simulink model "SupervisorB1"  (R2024b)
settings: Solver=FixedStepDiscrete  StartTime=0.0  StopTime=10.0  FixedStep=0.02  RelTol=1e-3
settings Model: DataDictionary=B1Sup.sldd  PacingRate=0.100000  Creator=miche  LastModifiedBy=Sterm
settings OptimizationCC: DefaultParameterBehavior=Inlined  EnhancedBackFolding=on  PassReuseOutputArgsAs=Individual arguments  ZeroExternalMemoryAtStartup=off  ZeroInternalMemoryAtStartup=off  OptimizeBlockOrder=speed  DifferentSizesBufferReuse=on  OptimizationCustomize=off  EfficientTunableParamExpr=on
settings DebuggingCC: ParameterTunabilityLossMsg=error
settings SFSimCC: MATLABDynamicMemAlloc=off
settings SFSimCC: SimUserIncludeDirs=|
  | C:\Users\Sterm\Desktop\STM32\workspace\Codice_Rover
  | C:\Users\Sterm\Desktop\STM32\workspace\Codice_Rover\Progetto_Board1\Core\Inc
settings RTWCC: Description=Embedded Coder  SystemTargetFile=ert.tlc  GenCodeOnly=on  TemplateMakefile=ert_default_tmf
settings CodeAppCC: ForceParamTrailComments=on  IgnoreCustomStorageClasses=off  OperatorAnnotations=on  SimulinkDataObjDesc=on  SFDataObjDesc=on  InsertBlockDesc=on
settings ERTTargetCC: TargetLangStandard=C99 (ISO)  GenerateSampleERTMain=on  ERTCustomFileTemplate=example_file_process.tlc

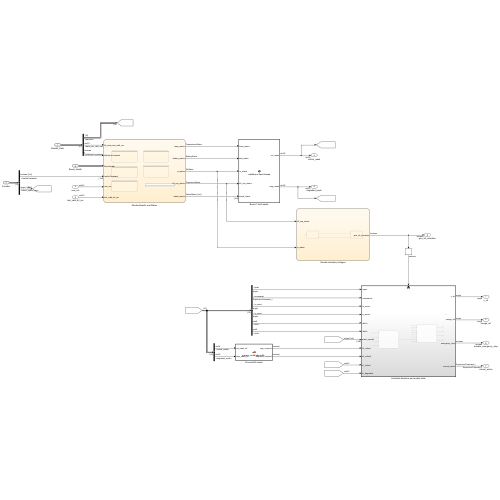
[thumbnail: Simulink's stored preview of the top-level diagram]
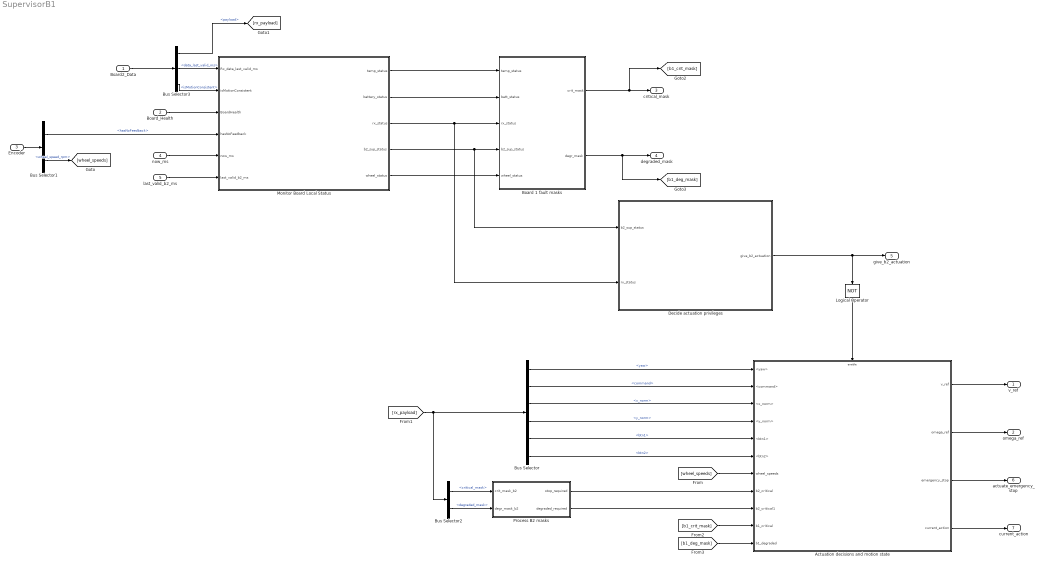
== system SupervisorB1 ==
  Board2_Data : Inport  OutDataTypeStr=Bus: RxSnapshot_t
  Board_Health : Inport  Port=2  OutDataTypeStr=Bus: BoardHealthSnapshot_t
  Encoder : Inport  Port=3  OutDataTypeStr=Bus: EncoderSnapshot_t
  now_ms : Inport  Port=4  OutDataTypeStr=uint32
  last_valid_b2_ms : Inport  Port=5  OutDataTypeStr=uint32
  Actuation decisions and motion state : Subsystem
  Board 1 fault masks : MATLAB Function  TreatAsAtomicUnit=on
  Bus Selector : BusSelector  OutputSignals=yaw,command,x_norm,y_norm,btn1,btn2
  Bus Selector1 : BusSelector  OutputSignals=hasNoFeedback,wheel_speed_rpm
  Bus Selector2 : BusSelector  OutputSignals=critical_mask,degraded_mask
  Bus Selector3 : BusSelector  OutputSignals=payload,data_last_valid_ms,payload.isMotionConsistent
  Decide actuation privileges : Stateflow chart  TreatAsAtomicUnit=on
      settings: RTWFcnNameOpts=Use subsystem name  RTWFileNameOpts=Use subsystem name  PortSchema="{\"entries\":[{\"content\":{\"sides\":[{\"content\":{\"connectorIds\":[\"In2\",\"In1\"]},\"type\":\"ConnectorPlacement.EquallySpacedRectSide\",\"uuid\":\"67b49e78-6b94-400e-9fcc-b30b67a80691\"},{\"content\":{\"connectorIds\":[\"Out1\"],\"side\":\"RIGHT\"},\"type\":\"ConnectorPlacement.EquallySpacedRectSide\",\"uuid\":\"f9efb856-d575-4b84-9867-a72704ddd64e\"},{\"content\":{\"side\":\"TOP\"},\"type\":\"ConnectorPlacement.EquallySpacedRectSide\",\"uuid\":\"fb0179cd-4de4-48aa-8472-d7b382cb3b22\"}]},\"type\":\"ConnectorPlacement.EquallySpacedConnector\",\"uuid\":\"a3077d23-e6fe-47c9-9a8f-de3eab952316\"}],\"packageUris\":[\"http://schema.mathworks.com/mf0/Connector/R2020b\"],\"version\":\"1.0\"}"
  Logical Operator : Logic  Operator=NOT  AllPortsSameDT=off  OutDataTypeStr=boolean
  Monitor Board Local Status : Stateflow chart  TreatAsAtomicUnit=on
      settings: PortSchema="{\"entries\":[{\"content\":{\"sides\":[{\"content\":{\"connectorIds\":[\"In2\",\"In5\",\"In1\",\"In4\",\"In3\",\"In6\"]},\"type\":\"ConnectorPlacement.EquallySpacedRectSide\",\"uuid\":\"47aaac17-a3c1-4cfa-9019-2fc909ce8afb\"},{\"content\":{\"connectorIds\":[\"Out1\",\"Out2\",\"Out3\",\"Out5\",\"Out4\"],\"side\":\"RIGHT\"},\"type\":\"ConnectorPlacement.EquallySpacedRectSide\",\"uuid\":\"50480d75-ffb6-4b14-98f4-247cb8499fa0\"},{\"content\":{\"side\":\"TOP\"},\"type\":\"ConnectorPlacement.EquallySpacedRectSide\",\"uuid\":\"1cb4b11b-b488-43f8-b4d2-41a29965dbbd\"}]},\"type\":\"ConnectorPlacement.EquallySpacedConnector\",\"uuid\":\"f85d8103-6e2e-468d-83b6-a974a06ba402\"}],\"packageUris\":[\"http://schema.mathworks.com/mf0/Connector/R2020b\"],\"version\":\"1.0\"}"
  Process B2 masks : MATLAB Function  TreatAsAtomicUnit=on
  v_ref : Outport  OutDataTypeStr=single
  omega_ref : Outport  Port=2  OutDataTypeStr=single
  critical_mask : Outport  Port=3  OutDataTypeStr=uint32
  degraded_mask : Outport  Port=4  OutDataTypeStr=uint32
  give_b2_actuation : Outport  Port=5  OutDataTypeStr=boolean
  actuate_emergency_stop : Outport  Port=6  OutDataTypeStr=boolean
  current_action : Outport  Port=7  OutDataTypeStr=Enum: SupervisorCommand_t
  wires:
  Board_Health/1 -> Monitor Board Local Status/1(BoardHealth)
  Encoder/1 -> Bus Selector1/1
  Board2_Data/1 -> Bus Selector3/1
  now_ms/1 -> Monitor Board Local Status/3(now_ms)
  Board 1 fault masks/2(degr_mask) -> [b1_deg_mask], degraded_mask/1
  Board 1 fault masks/1(crit_mask) -> [b1_crit_mask], critical_mask/1
  Bus Selector1/1 -> Monitor Board Local Status/4(hasNoFeedback)  "<hasNoFeedback>"
  Monitor Board Local Status/1(temp_status) -> Board 1 fault masks/1(temp_status)
  Monitor Board Local Status/2(battery_status) -> Board 1 fault masks/2(batt_status)
  Monitor Board Local Status/4(wheel_status) -> Board 1 fault masks/5(wheel_status)
  last_valid_b2_ms/1 -> Monitor Board Local Status/6(last_valid_b2_ms)
  Bus Selector3/2 -> Monitor Board Local Status/2(Rx_data_last_valid_ms)  "<data_last_valid_ms>"
  Monitor Board Local Status/3(rx_status) -> Decide actuation privileges/1(rx_status), Board 1 fault masks/3(rx_status)
  Monitor Board Local Status/5(b2_sup_status) -> Decide actuation privileges/2(b2_sup_status), Board 1 fault masks/4(b2_sup_status)
  Decide actuation privileges/1(give_b2_actuation) -> give_b2_actuation/1, Logical Operator/1
  Bus Selector1/2 -> [wheel_speeds]  "<wheel_speed_rpm>"
  Bus Selector/2 -> Actuation decisions and motion state/2(<command>)  "<command>"
  Bus Selector/1 -> Actuation decisions and motion state/1(<yaw>)  "<yaw>"
  [wheel_speeds] -> Actuation decisions and motion state/7(wheel_speeds)
  Bus Selector/3 -> Actuation decisions and motion state/3(<x_norm>)  "<x_norm>"
  Bus Selector/4 -> Actuation decisions and motion state/4(<y_norm>)  "<y_norm>"
  Bus Selector/5 -> Actuation decisions and motion state/5(<btn1>)  "<btn1>"
  Bus Selector/6 -> Actuation decisions and motion state/6(<btn2>)  "<btn2>"
  Actuation decisions and motion state/2(omega_ref) -> omega_ref/1
  Actuation decisions and motion state/1(v_ref) -> v_ref/1
  Actuation decisions and motion state/3(emergency_stop) -> actuate_emergency_stop/1
  Actuation decisions and motion state/4(current_action) -> current_action/1
  Process B2 masks/1(stop_required) -> Actuation decisions and motion state/8(b2_critical)
  Process B2 masks/2(degraded_required) -> Actuation decisions and motion state/9(b2_critical1)
  Bus Selector3/1 -> [rx_payload]  "<payload>"
  Bus Selector3/3 -> Monitor Board Local Status/5(isMotionConsistent)  "<isMotionConsistent>"
  Logical Operator/1 -> Actuation decisions and motion state/Enable
  [b1_crit_mask] -> Actuation decisions and motion state/10(b1_critical)
  [b1_deg_mask] -> Actuation decisions and motion state/11(b1_degraded)
  [rx_payload] -> Bus Selector2/1, Bus Selector/1
  Bus Selector2/1 -> Process B2 masks/1(crit_mask_b2)  "<critical_mask>"
  Bus Selector2/2 -> Process B2 masks/2(degr_mask_b2)  "<degraded_mask>"

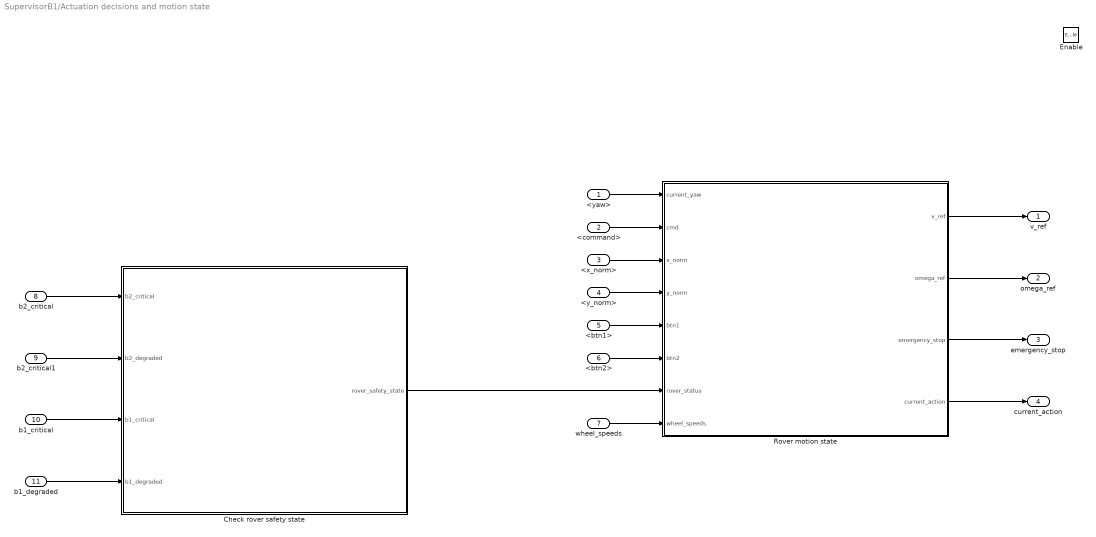
== system SupervisorB1/Actuation decisions and motion state ==
  <yaw> : Inport
  <command> : Inport  Port=2
  <x_norm> : Inport  Port=3
  <y_norm> : Inport  Port=4
  <btn1> : Inport  Port=5
  <btn2> : Inport  Port=6
  wheel_speeds : Inport  Port=7
  b2_critical : Inport  Port=8
  b2_critical1 : Inport  Port=9
  b1_critical : Inport  Port=10
  b1_degraded : Inport  Port=11
  Enable : EnablePort
  Check rover safety state : Stateflow chart  TreatAsAtomicUnit=on
      settings: PortSchema="{\"entries\":[{\"content\":{\"sides\":[{\"content\":{\"connectorIds\":[\"In3\",\"In4\",\"In1\",\"In2\"]},\"type\":\"ConnectorPlacement.EquallySpacedRectSide\",\"uuid\":\"9dc33dbe-e010-4406-a301-8909eb6c65d2\"},{\"content\":{\"connectorIds\":[\"Out1\"],\"side\":\"RIGHT\"},\"type\":\"ConnectorPlacement.EquallySpacedRectSide\",\"uuid\":\"084d7bfb-fdfa-425b-9b48-9ea13f8992e6\"},{\"content\":{\"side\":\"TOP\"},\"type\":\"ConnectorPlacement.EquallySpacedRectSide\",\"uuid\":\"e02a7452-bac4-4562-b32b-e5d8b54b8354\"}]},\"type\":\"ConnectorPlacement.EquallySpacedConnector\",\"uuid\":\"22e5b97d-2191-437a-a89c-d8bb13bb1f1c\"}],\"packageUris\":[\"http://schema.mathworks.com/mf0/Connector/R2020b\"],\"version\":\"1.0\"}"
  Rover motion state : Stateflow chart  TreatAsAtomicUnit=on
      settings: PortSchema="{\"entries\":[{\"content\":{\"sides\":[{\"content\":{\"connectorIds\":[\"In2\",\"In1\",\"In4\",\"In5\",\"In7\",\"In8\",\"In6\",\"In3\"]},\"type\":\"ConnectorPlacement.EquallySpacedRectSide\",\"uuid\":\"ab2cffc6-18c1-4b62-a79f-6b348f0e6e12\"},{\"content\":{\"connectorIds\":[\"Out2\",\"Out1\",\"Out3\",\"Out4\"],\"side\":\"RIGHT\"},\"type\":\"ConnectorPlacement.EquallySpacedRectSide\",\"uuid\":\"a6f1ea66-886a-456c-a684-893d1155cc5f\"},{\"content\":{\"side\":\"TOP\"},\"type\":\"ConnectorPlacement.EquallySpacedRectSide\",\"uuid\":\"8507e94f-e138-4434-ac51-1bc550838c0e\"}]},\"type\":\"ConnectorPlacement.EquallySpacedConnector\",\"uuid\":\"3184930e-9ebc-43d7-b63a-062e80318630\"}],\"packageUris\":[\"http://schema.mathworks.com/mf0/Connector/R2020b\"],\"version\":\"1.0\"}"
  v_ref : Outport
  omega_ref : Outport  Port=2
  emergency_stop : Outport  Port=3
  current_action : Outport  Port=4
  wires:
  wheel_speeds/1 -> Rover motion state/3(wheel_speeds)
  Rover motion state/2(v_ref) -> v_ref/1
  <command>/1 -> Rover motion state/1(cmd)
  <y_norm>/1 -> Rover motion state/5(y_norm)
  <btn2>/1 -> Rover motion state/8(btn2)
  Rover motion state/1(omega_ref) -> omega_ref/1
  Rover motion state/3(emergency_stop) -> emergency_stop/1
  Rover motion state/4(current_action) -> current_action/1
  <x_norm>/1 -> Rover motion state/4(x_norm)
  <yaw>/1 -> Rover motion state/2(current_yaw)
  <btn1>/1 -> Rover motion state/7(btn1)
  Check rover safety state/1(rover_safety_state) -> Rover motion state/6(rover_status)
  b1_critical/1 -> Check rover safety state/1(b1_critical)
  b2_critical/1 -> Check rover safety state/3(b2_critical)
  b1_degraded/1 -> Check rover safety state/2(b1_degraded)
  b2_critical1/1 -> Check rover safety state/4(b2_degraded)

== stateflow chart SupervisorB1/Monitor Board Local Status ==
  state MonitorTemperature [parallel]
    settings: executionOrder=1
    state Temperature_timeout
      en:
      temp_status = TEMP_HEALTH_CRITICAL;
    state Temperature_ok
      en:
      temp_status = TEMP_HEALTH_OK;
    state Temperature_degraded
      en:
      temp_status = TEMP_HEALTH_DEGRADED;
    state Temperature_critical
      en:
      temp_status = TEMP_HEALTH_CRITICAL;
    Temperature_timeout -> (junction 473) : [duration(BoardHealth.temperature_degC < 50 || BoardHealth.temperature_degC > 0) > 5]
    (junction 473) -> Temperature_ok
    (junction 474) -> Temperature_timeout
    (junction 475) -> Temperature_timeout
    Temperature_ok -> (junction 474) [order 2] : [checkTempTimeout(now_ms, BoardHealth.temp_last_valid_ms, ...
        |     BoardHealth.temperature_degC)]
    Temperature_degraded -> (junction 475) [order 3] : [checkTempTimeout(now_ms, BoardHealth.temp_last_valid_ms, ...
        |     BoardHealth.temperature_degC)]
    Temperature_degraded -> Temperature_ok [order 1] : [duration(BoardHealth.temperature_degC < 50 || BoardHealth.temperature_degC > 0) > 10]
    (default) -> Temperature_ok
    Temperature_ok -> Temperature_degraded [order 1] : [duration(BoardHealth.temperature_degC > 55 || BoardHealth.temperature_degC < -5) > 10]
    (junction 476) -> Temperature_ok : [duration(BoardHealth.temperature_degC < 50 || BoardHealth.temperature_degC > 0) > 5]
    Temperature_degraded -> (junction 477) [order 2] : [duration(BoardHealth.temperature_degC > 65 || BoardHealth.temperature_degC < -15) > 4]
    Temperature_critical -> (junction 476)
    (junction 477) -> Temperature_critical
  state MonitorBattery [parallel]
    settings: executionOrder=2
    state Battery_timeout
      en:
      battery_status = BATTERY_HEALTH_CRITICAL;
    state Battery_ok
      en:
      battery_status = BATTERY_HEALTH_OK;
    state Battery_degraded
      en:
      battery_status = BATTERY_HEALTH_DEGRADED;
    state Battery_critical
      en:
      battery_status = BATTERY_HEALTH_CRITICAL;
    Battery_timeout -> (junction 527) : [duration(BoardHealth.battery_pct > 25) > 5]
    (junction 527) -> Battery_ok
    (junction 528) -> Battery_timeout
    (junction 529) -> Battery_timeout
    Battery_ok -> (junction 528) [order 2] : [checkBatteryTimeout(now_ms,BoardHealth.batt_last_valid_ms, BoardHealth.battery_pct)]
    Battery_degraded -> (junction 529) [order 3] : [checkBatteryTimeout(now_ms,BoardHealth.batt_last_valid_ms, BoardHealth.battery_pct)]
    Battery_degraded -> Battery_ok [order 1] : [duration(BoardHealth.battery_pct > 25) > 5]
    (default) -> Battery_ok
    Battery_ok -> Battery_degraded [order 1] : [duration(BoardHealth.battery_pct < 23) > 5]
    (junction 530) -> Battery_ok : [duration(BoardHealth.battery_pct > 25) > 5]
    Battery_degraded -> (junction 531) [order 2] : [duration(BoardHealth.battery_pct < 15) > 5]
    Battery_critical -> (junction 530)
    (junction 531) -> Battery_critical
  state MonitorWheels [parallel]
    settings: executionOrder=3
    state MonitorFrontLeft [parallel]
      settings: executionOrder=1
      state FrontLeft_motor_critical
        en:
        wheel_status(1) = WHEEL_CRITICAL_MOTOR;
      state FrontLeft_ok
        en:
        wheel_status(1) = WHEEL_OK;
      state FrontLeft_encoder_critical
        en:
        wheel_status(1) = WHEEL_DEGRADED_ENCODER;
      (junction 622) -> FrontLeft_motor_critical
      FrontLeft_encoder_critical -> (junction 622) [order 2] : [~isMotionConsistent && rx_status ~= RX_CRITICAL]
      FrontLeft_encoder_critical -> FrontLeft_ok [order 1] : [~hasNoFeedback(1)]
      (default) -> FrontLeft_ok
      FrontLeft_ok -> FrontLeft_encoder_critical : [hasNoFeedback(1)]
    state MonitorFrontRight [parallel]
      settings: executionOrder=2
      state FrontRight_motor_critical
        en:
        wheel_status(2) = WHEEL_CRITICAL_MOTOR;
      state FrontRight_ok
        en:
        wheel_status(2) = WHEEL_OK;
      state FrontRight_encoder_critical
        en:
        wheel_status(2) = WHEEL_DEGRADED_ENCODER;
      (junction 652) -> FrontRight_motor_critical
      FrontRight_encoder_critical -> (junction 652) [order 2] : [~isMotionConsistent && rx_status ~= RX_CRITICAL]
      FrontRight_encoder_critical -> FrontRight_ok [order 1] : [~hasNoFeedback(2)]
      (default) -> FrontRight_ok
      FrontRight_ok -> FrontRight_encoder_critical : [hasNoFeedback(2)]
    state MonitorRearRight [parallel]
      settings: executionOrder=4
      state RearRight_motor_critical
        en:
        wheel_status(4) = WHEEL_CRITICAL_MOTOR;
      state RearRight_ok
        en:
        wheel_status(4) = WHEEL_OK;
      state RearRight_encoder_critical
        en:
        wheel_status(4) = WHEEL_DEGRADED_ENCODER;
      (junction 672) -> RearRight_motor_critical
      RearRight_encoder_critical -> (junction 672) [order 2] : [~isMotionConsistent && rx_status ~= RX_CRITICAL]
      RearRight_encoder_critical -> RearRight_ok [order 1] : [~hasNoFeedback(4)]
      (default) -> RearRight_ok
      RearRight_ok -> RearRight_encoder_critical : [hasNoFeedback(4)]
    state MonitorRearLeft [parallel]
      settings: executionOrder=3
      state RearLeft_motor_critical
        en:
        wheel_status(3) = WHEEL_CRITICAL_MOTOR;
      state RearLeft_ok
        en:
        wheel_status(3) = WHEEL_OK;
      state RearLeft_encoder_critical
        en:
        wheel_status(3) = WHEEL_DEGRADED_ENCODER;
      (junction 662) -> RearLeft_motor_critical
      RearLeft_encoder_critical -> (junction 662) [order 2] : [~isMotionConsistent && rx_status ~= RX_CRITICAL]
      RearLeft_encoder_critical -> RearLeft_ok [order 1] : [~hasNoFeedback(3)]
      (default) -> RearLeft_ok
      RearLeft_ok -> RearLeft_encoder_critical : [hasNoFeedback(3)]
  state MonitorBoard2Supervisor [parallel]
    settings: executionOrder=4
    state B2_sup_critical
      en:
      b2_sup_status = SUPERVISOR_CRITICAL;
      du:
      degraded_sup = isCommDegradedByMeanPeriod(...
      last_valid_b2_ms, 40);
    state B2_sup_ok
      en:
      b2_sup_status = SUPERVISOR_OK;
      du:
      degraded_sup = isCommDegradedByMeanPeriod(...
      last_valid_b2_ms, 40);
    state B2_sup_degraded
      en:
      b2_sup_status = SUPERVISOR_DEGRADED;
      du:
      degraded_sup = isCommDegradedByMeanPeriod(...
      last_valid_b2_ms, 40);
    B2_sup_critical -> (junction 713) : [duration(~degraded_sup) > 1]
    (junction 713) -> B2_sup_ok
    (junction 712) -> B2_sup_critical
    (junction 717) -> B2_sup_critical
    B2_sup_ok -> (junction 712) [order 2] : [now_ms - last_valid_b2_ms > 120]
    B2_sup_degraded -> (junction 717) [order 2] : [now_ms - last_valid_b2_ms > 120]
    B2_sup_degraded -> B2_sup_ok [order 1] : [duration(~degraded_sup) > 1]
    (default) -> B2_sup_ok
    B2_sup_ok -> B2_sup_degraded [order 1] : [degraded_sup]
  state MonitorRx [parallel]
    settings: executionOrder=5
    state Rx_critical
      en:
      rx_status = RX_CRITICAL;
      du:
      degraded_rx = isCommDegradedByMeanPeriod(...
      Rx_data_last_valid_ms, 40);
    state Rx_ok
      en:
      rx_status = RX_OK;
      du:
      degraded_rx = isCommDegradedByMeanPeriod(...
      Rx_data_last_valid_ms, 40);
    state Rx_degraded
      en:
      rx_status = RX_DEGRADED;
      du:
      degraded_rx = isCommDegradedByMeanPeriod(...
      Rx_data_last_valid_ms, 40);
    Rx_critical -> (junction 732) : [duration(~degraded_rx) > 1]
    (junction 732) -> Rx_ok
    (junction 733) -> Rx_critical
    (junction 734) -> Rx_critical
    Rx_ok -> (junction 733) [order 2] : [now_ms - Rx_data_last_valid_ms > 120]
    Rx_degraded -> (junction 734) [order 2] : [now_ms - Rx_data_last_valid_ms > 120]
    Rx_degraded -> Rx_ok [order 1] : [duration(~degraded_rx) > 1]
    (default) -> Rx_ok
    Rx_ok -> Rx_degraded [order 1] : [degraded_rx]
  data: now_ms function_input; temp_last_valid_ms function_input; temperature_degC function_input; timeout_fault function_output; now_ms function_input; batt_last_valid_ms function_input; batt_pct_last function_input; timeout_fault function_output; data_last_valid_ms function_input; mean_threshold_ms function_input; comm_degraded function_output; BoardHealth input Bus: BoardHealthSnapshot_t; Rx_data_last_valid_ms input; temp_status output Enum: TemperatureStatus; battery_status output Enum: BatteryStatus; rx_status output Enum: RxStatus =RxStatus.RX_OK; now_ms input; hasNoFeedback input boolean size=[1 4]; isMotionConsistent input boolean; wheel_status output Enum: WheelStatus size=[1 4]; last_valid_b2_ms input; b2_sup_status output Enum: SupervisorStatus; degraded_rx local =false; degraded_sup local =false
  function timeout_fault = checkTempTimeout( ...:
    | function timeout_fault = checkTempTimeout( ...
    |     now_ms, ...
    |     temp_last_valid_ms, ...
    |     temperature_degC)
    | 
    | % CHECKTEMPTIMEOUT
    | % Valuta se un timeout della misura temperatura è pericoloso
    | % usando una stima worst-case della crescita termica.
    | %
    | % INPUT:
    | %   now_ms                 timestamp corrente [ms]
    | %   temp_last_valid_ms     timestamp ultimo dato valido [ms]
    | %   temperature_degC       ultima temperatura valida [°C]
    | %
    | % OUTPUT:
    | %   timeout_fault          true  -> attiva fault / safe stop
    | %                           false -> ok (non pericoloso)
    | 
    |     % ----------------------------
    |     % PARAMETRI DI PROGETTO
    |     % ----------------------------
    |     T_fault = 65;        % °C  (limite STM32)
    |     r_max   = single(1.0);       % °C/s worst-case crescita
    |     t_min   = single(0.5);       % s   ignora timeout troppo brevi (rumore)
    | 
    |     % ----------------------------
    |     % CALCOLO TIMEOUT
    |     % ----------------------------
    |     dt_ms = now_ms - temp_last_valid_ms;
    | 
    |     dt_s = dt_ms / 1000.0;
    | 
    |     % Se il timeout è troppo breve, non è pericoloso
    |     if dt_s < t_min
    |         timeout_fault = false;
    |         return;
    |     end
    | 
    |     % ----------------------------
    |     % WORST-CASE TEMPERATURA
    |     % ----------------------------
    |     T_worst = temperature_degC + r_max * single(dt_s);
    | 
    |     % ----------------------------
    |     % DECISIONE
    |     % ----------------------------
    |     timeout_fault = (T_worst >= T_fault);
    | 
    | end
  function timeout_fault = checkBatteryTimeout( ...:
    | function timeout_fault = checkBatteryTimeout( ...
    |     now_ms, ...
    |     batt_last_valid_ms, ...
    |     batt_pct_last)
    | 
    | % CHECKBATTERYTIMEOUT
    | % Valuta se la perdita della misura batteria è pericolosa
    | % usando una stima worst-case di scarica.
    | %
    | % INPUT:
    | %   now_ms               timestamp corrente [ms]
    | %   batt_last_valid_ms   timestamp ultimo dato valido [ms]
    | %   batt_pct_last        ultima percentuale valida [%]
    | %
    | % OUTPUT:
    | %   timeout_fault        true  -> fault / stop
    | %                         false -> ok
    | 
    |     % ----------------------------
    |     % PARAMETRI DI PROGETTO
    |     % ----------------------------
    |     SOC_fault = 23;          % % soglia di fault
    |     C_nom_Ah  = 3.3;         % Ah capacità batteria
    |     I_max     = 50.0;        % A worst-case consumo totale
    |     t_min     = 0.5;         % s ignora timeout brevissimi
    | 
    |     %Il worst case presuppone che vengano consumati 0.42% di batteria al
    |     %secondo, quindi se arrivo a 30% e aspetto per 5 secondi che sia
    |     %costante allora può scendere massimo a circa 27/28%, questo mi
    |     %permette di ridurre il rumore di misura senza scendere
    |     %inavvertitamente sotto la soglia di fault (23%)
    |     
    |     % ----------------------------
    |     % TEMPO TRASCORSO
    |     % ----------------------------
    |     dt_ms = now_ms - batt_last_valid_ms;
    |     dt_s  = dt_ms / 1000.0;
    | 
    |     if dt_s < t_min
    |         timeout_fault = false;
    |         return;
    |     end
    | 
    |     % ----------------------------
    |     % WORST-CASE SCARICA
    |     % ----------------------------
    |     % Ah consumati nel worst-case
    |     Ah_used = I_max * (dt_s / 3600.0);
    | 
    |     % Conversione in percentuale
    |     soc_drop = single((Ah_used / C_nom_Ah) * 100.0);
    | 
    |     soc_worst = batt_pct_last - soc_drop;
    | 
    |     % ----------------------------
    |     % DECISIONE
    |     % ----------------------------
    |     timeout_fault = (soc_worst <= SOC_fault);
    | 
    | end
  function comm_degraded = isCommDegradedByMeanPeriod(data_last_valid_ms, mean_threshold_ms):
    | function comm_degraded = isCommDegradedByMeanPeriod(data_last_valid_ms, mean_threshold_ms)
    | % ISCOMMDEGRADEDBYMEANPERIOD
    | % Valuta stato "degraded" in base alla media dei tempi di arrivo dati.
    | %
    | % INPUT:
    | %   data_last_valid_ms   - timestamp ultimo dato valido (ms)
    | %   mean_threshold_ms    - soglia media periodo (ms), es. 100
    | %
    | % OUTPUT:
    | %   comm_degraded        - true se mean_dt > mean_threshold_ms
    | %   mean_dt              - periodo medio stimato (ms)
    | 
    | % ----------------------------
    | % PARAMETRI DI PROGETTO
    | % ----------------------------
    | N_SAMPLES = 10;   % numero di periodi mediati
    | 
    | % ----------------------------
    | % STATO PERSISTENTE
    | % ----------------------------
    | persistent last_valid_prev buf idx count sum_dt
    | 
    | if isempty(last_valid_prev)
    |     last_valid_prev = data_last_valid_ms;
    |     buf   = zeros(1, N_SAMPLES);
    |     idx   = 1;
    |     count = 0;
    |     sum_dt = uint32(0);
    | 
    |     comm_degraded = false;
    |     return;
    | end
    | 
    | % ----------------------------
    | % NUOVO DATO ARRIVATO?
    | % ----------------------------
    | if data_last_valid_ms ~= last_valid_prev
    | 
    |     dt = data_last_valid_ms - last_valid_prev;
    |     last_valid_prev = data_last_valid_ms;
    | 
    |     % Sliding window O(1)
    |     old = buf(idx);
    |     buf(idx) = dt;
    |     sum_dt = sum_dt - old + dt;
    | 
    |     idx = idx + 1;
    |     if idx > N_SAMPLES
    |         idx = 1;
    |     end
    | 
    |     if count < N_SAMPLES
    |         count = count + 1;
    |     end
    | end
    | 
    | % ----------------------------
    | % MEDIA E DECISIONE
    | % ----------------------------
    | if count > 0
    |     mean_dt = sum_dt / count;
    | else
    |     mean_dt = uint32(0);
    | end
    | 
    | comm_degraded = (mean_dt > mean_threshold_ms);
    | 
    | end

== stateflow chart SupervisorB1/Actuation decisions and motion state/Rover motion state ==
  state Backward_mode_toggle [parallel]
    settings: executionOrder=1
    state Combo_toggle_backward
      state Step2
      state Step3
      state Step4
      Step2 -> Step3 [order 1] : [ rising(btn1)]
      Step2 -> (junction 901) [order 2] : [after(1,sec)]
      Step3 -> (junction 901) [order 2] : [after(1,sec)]
      Step3 -> Step4 [order 1] : [rising(btn2)]
      Step4 -> (junction 901) [order 2] : [after(1,sec)]
    state Combo_starting_point
    Combo_starting_point -> Step2 : [rising(btn1) && x_norm == 0 && y_norm == 0]
    (default) -> Combo_starting_point : {backward_enabled = false;}
    Combo_toggle_backward -> Combo_starting_point : [x_norm ~= 0 || y_norm ~= 0]
    (junction 901) -> Combo_starting_point
    (junction 907) -> Combo_starting_point
    Step4 -> (junction 906) [order 1] : [rising(btn2)]
    (junction 906) -> (junction 907) : {backward_enabled = ~backward_enabled}
  state Motion_Supervision [parallel]
    settings: executionOrder=2
    state Stato_marcia_rover
      en,du:
      [V_MAX, OMEGA_MAX, V_MAX_MANEUVER, OMEGA_GO_LEFT, OMEGA_GO_RIGHT] = updateSafetyLimits(rover_status);
      v_user     = y_norm * V_MAX;
      omega_user = x_norm * OMEGA_MAX;
      if invert_y
      if v_user >= 0
      invert_y = false;
      else
      v_user = -v_user;
      end
      end
      ex:
      invert_y = false;
      state Evita_destra
        en:
        current_action = CMD_AVOID_RIGHT;
        du:
        v_ref = v_user;
        omega_ref = max(omega_user, 0);
      state Evita_sinistra
        en:
        current_action = CMD_AVOID_LEFT;
        du:
        v_ref = v_user;
        omega_ref = min(omega_user, 0);
      state Schivata_a_sinistra
        en:
        current_action = CMD_GO_LEFT;
        du:
        v_ref = min(v_user, V_MAX_MANEUVER);
        omega_ref = max(omega_user, OMEGA_GO_LEFT);
      state Normale_marcia
        en:
        current_action = CMD_NORMAL;
        du:
        if backward_enabled || y_norm > 0
        v_ref = v_user;
        omega_ref = omega_user;
        else
        v_ref = 0;
        omega_ref = omega_user;
        end
      state Schivata_a_destra
        en:
        current_action = CMD_GO_RIGHT;
        du:
        v_ref = min(v_user, V_MAX_MANEUVER);
        omega_ref = min(omega_user, OMEGA_GO_RIGHT);
      state Retromarcia_180
        en:
        current_action = CMD_ROTATE_180;
        is_rotating180 = true;
        targetAngle = angleCalculator180(current_yaw);
        angle_err = angleError(current_yaw, targetAngle)
        du:
        angle_err = angleError(current_yaw, targetAngle)
        if abs(angle_err) > 45
        omega_ref = sign(-angle_err) *OMEGA_MAX;
        elseif rover_status == SAFETY_OK
        omega_ref = sign(-angle_err) * min(OMEGA_MAX, max(abs(angle_err),15) * 0.005);
        end
        ex:
        is_rotating180 = false;
      Normale_marcia -> Evita_destra [order 3] : [v_user > 0 && cmd == CMD_AVOID_RIGHT]
      Evita_destra -> Normale_marcia : [cmd == CMD_NORMAL]
      Evita_sinistra -> Normale_marcia : [cmd == CMD_NORMAL]
      Normale_marcia -> Evita_sinistra [order 2] : [v_user > 0 && cmd == CMD_AVOID_LEFT]
      Schivata_a_sinistra -> Normale_marcia : [cmd == CMD_NORMAL]
      Schivata_a_destra -> Normale_marcia : [cmd == CMD_NORMAL]
      Normale_marcia -> Schivata_a_destra [order 4] : [v_user >0 && cmd == CMD_GO_RIGHT]
      Normale_marcia -> Schivata_a_sinistra [order 1] : [v_user > 0 && cmd == CMD_GO_LEFT]
      (default) -> Normale_marcia
      (junction 1022) -> Normale_marcia
      (junction 1056) -> (junction 1022)
      (junction 1055) -> (junction 1022) [order 2]
      Normale_marcia -> Retromarcia_180 [order 5] : [y_norm < -0.5 && ~backward_enabled]
      Retromarcia_180 -> (junction 1055) : [abs(angle_err) < 7.5]
      (junction 1055) -> (junction 1056) [order 1] : [v_user < 0]
          | {invert_y = true;}
    state Procedura_emergency_stop
      state In_frenata_di_emergenza
        en:
        current_action = CMD_ESTOP;
        v_ref = 0;
        omega_ref = 0;
        emergency_stop = true;
        du:
        roverIsStopped = checkStop(wheel_speeds)
      state Motori_fermi
        en:
        current_action = CMD_STOP;
        estop_recover_enabled = true;
      In_frenata_di_emergenza -> Motori_fermi : [duration(roverIsStopped) > 1]
    Stato_marcia_rover -> In_frenata_di_emergenza : [(cmd == CMD_ESTOP && v_user > 0 && ~is_rotating180) || rover_status == SAFETY_CRITICAL]
        | {
        | estop_recover_enabled = false;
        | }
    (default) -> Stato_marcia_rover
    Procedura_emergency_stop -> Stato_marcia_rover : [rover_status ~= SAFETY_CRITICAL && estop_recover_enabled]
        | {
        | emergency_stop = false;
        | }
  data: gyro_angle function_input; targetAngle function_input; angle_err function_output; gyro_angle function_input; targetAngle function_output; rover_state function_input; V_MAX function_output; OMEGA_MAX function_output; V_MAX_MANEUVER function_output; OMEGA_GO_LEFT function_output; OMEGA_GO_RIGHT function_output; wheel_speeds function_input; stop function_output; cmd input Enum: SupervisorCommand_t; current_yaw input; wheel_speeds input; omega_ref output; angle_err local; roverIsStopped local =false; x_norm input; y_norm input; OMEGA_GO_LEFT local; OMEGA_GO_RIGHT local; OMEGA_MAX local; V_MAX local; V_MAX_MANEUVER local; is_rotating180 local; v_user local; omega_user local; v_ref output; rover_status input Enum: SafetyStatus; invert_y local; emergency_stop output; current_action output Enum: SupervisorCommand_t; estop_recover_enabled local; btn1 input; btn2 input; backward_enabled local; targetAngle local
  function angle_err = angleError(gyro_angle, targetAngle):
    | function angle_err = angleError(gyro_angle, targetAngle)
    |     % errore in gradi, range [-180, +180]
    |     angle_err = mod(targetAngle - gyro_angle + 180, 360) - 180;
    | end
  function targetAngle = angleCalculator180(gyro_angle):
    | function targetAngle = angleCalculator180(gyro_angle)
    | 
    |     angle = gyro_angle + 180;
    |     if angle > 360
    |         targetAngle = angle - 360;
    |     else
    |         targetAngle = angle;
    |     end
    | end
  function [V_MAX, OMEGA_MAX, V_MAX_MANEUVER, OMEGA_GO_LEFT, OMEGA_GO_RIGHT] = ...:
    | function [V_MAX, OMEGA_MAX, V_MAX_MANEUVER, OMEGA_GO_LEFT, OMEGA_GO_RIGHT] = ...
    |          updateSafetyLimits(rover_state)
    | 
    | % ---- valori nominali ----
    | V_MAX          = 1.0;
    | OMEGA_MAX      = 1.0;
    | V_MAX_MANEUVER = 0.8;
    | OMEGA_GO_LEFT  = 0.4;
    | OMEGA_GO_RIGHT = -0.4;
    | 
    | % ---- scaling in base allo stato ----
    | if rover_state == SafetyStatus.SAFETY_DEGRADED
    | 
    |     V_MAX          = 0.5 * V_MAX;
    |     OMEGA_MAX      = 0.5 * OMEGA_MAX;
    |     V_MAX_MANEUVER = 0.5 * V_MAX_MANEUVER;
    |     OMEGA_GO_LEFT  = 0.5 * OMEGA_GO_LEFT;
    |     OMEGA_GO_RIGHT = 0.5 * OMEGA_GO_RIGHT;
    | 
    | elseif rover_state == SafetyStatus.SAFETY_CRITICAL
    | 
    |     V_MAX          = 0;
    |     OMEGA_MAX      = 0;
    |     V_MAX_MANEUVER = 0;
    |     OMEGA_GO_LEFT  = 0;
    |     OMEGA_GO_RIGHT = 0;
    | 
    | end
    | 
    | end
  function stop = checkStop(wheel_speeds):
    | function stop = checkStop(wheel_speeds)
    | 
    | 
    | stop = all(abs(wheel_speeds(1:4)) < 2.5);
    | 
    | end

== stateflow chart SupervisorB1/Decide actuation privileges ==
  state B1_actuating
    en:
    give_b2_actuation = false;
  state B2_actuating
    en:
    give_b2_actuation = true;
  B1_actuating -> B2_actuating : [rx_status == RX_CRITICAL || b2_sup_status == SUPERVISOR_CRITICAL]
  (default) -> B1_actuating
  B2_actuating -> B1_actuating : [duration(rx_status ~= RX_CRITICAL && b2_sup_status ~= SUPERVISOR_CRITICAL) > 3]
  data: rx_status input Enum: RxStatus; give_b2_actuation output; b2_sup_status input Enum: SupervisorStatus

== stateflow chart SupervisorB1/Actuation decisions and motion state/Check rover safety state ==
  state Rover_Safe_State
    en:
    rover_safety_state = SAFETY_OK;
  state Rover_Degraded_State
    en:
    rover_safety_state = SAFETY_DEGRADED;
  state Rover_Critical_State
    en:
    rover_safety_state = SAFETY_CRITICAL;
  (junction 501) -> (junction 503) : [ ~(b1_degraded || b2_degraded)]
  (junction 503) -> Rover_Safe_State
  Rover_Degraded_State -> (junction 501) [order 1]
  Rover_Safe_State -> Rover_Degraded_State [order 2] : [b1_degraded || b2_degraded]
  (default) -> Rover_Safe_State
  (junction 476) -> Rover_Safe_State [order 1] : [~(b1_degraded || b2_degraded)]
  (junction 476) -> Rover_Degraded_State [order 2] : [b1_degraded || b2_degraded]
  Rover_Critical_State -> (junction 476) : [~(b1_critical || b2_critical)]
  Rover_Degraded_State -> (junction 506) [order 2]
  Rover_Safe_State -> (junction 481) [order 1] : [b1_critical || b2_critical]
  (junction 481) -> Rover_Critical_State
  (junction 506) -> Rover_Critical_State : [b1_critical || b2_critical]
  data: rover_safety_state output Enum: SafetyStatus; b1_critical input; b1_degraded input; b2_critical input; b2_degraded input

== matlab function SupervisorB1/Board 1 fault masks ==
  data: temp_status input; crit_mask output; batt_status input; rx_status input; b2_sup_status input; degr_mask output; wheel_status input
function [crit_mask, degr_mask] = buildBoard1FaultMasks( ...
    temp_status, batt_status, rx_status, b2_sup_status, wheel_status)

crit_mask = uint32(0);
degr_mask = uint32(0);

% ---- TEMPERATURA ----
if temp_status == TemperatureStatus.TEMP_HEALTH_CRITICAL
    crit_mask = bitor(crit_mask, bitshift(uint32(1), 0));
elseif temp_status == TemperatureStatus.TEMP_HEALTH_DEGRADED
    degr_mask = bitor(degr_mask, bitshift(uint32(1), 0));
end

% ---- BATTERIA ----
if batt_status == BatteryStatus.BATTERY_HEALTH_CRITICAL
    crit_mask = bitor(crit_mask, bitshift(uint32(1), 1));
elseif batt_status == BatteryStatus.BATTERY_HEALTH_DEGRADED
    degr_mask = bitor(degr_mask, bitshift(uint32(1), 1));
end

% ---- RX ----
if rx_status == RxStatus.RX_CRITICAL
    crit_mask = bitor(crit_mask, bitshift(uint32(1), 2));
elseif rx_status == RxStatus.RX_DEGRADED
    degr_mask = bitor(degr_mask, bitshift(uint32(1), 2));
end

% ---- WHEELS ----

for i = 1:4
    bit_idx = uint32(2 + i);  % FL=3, FR=4, RL=5, RR=6

    if wheel_status(i) == WheelStatus.WHEEL_CRITICAL_MOTOR
        crit_mask = bitor(crit_mask, bitshift(uint32(1), bit_idx));
    elseif wheel_status(i) == WheelStatus.WHEEL_DEGRADED_ENCODER
        degr_mask = bitor(degr_mask, bitshift(uint32(1), bit_idx));
    end
end


% ---- B2 supervisor ----
if b2_sup_status == SupervisorStatus.SUPERVISOR_CRITICAL
    crit_mask = bitor(crit_mask, bitshift(uint32(1), 7));
elseif b2_sup_status == SupervisorStatus.SUPERVISOR_DEGRADED
    degr_mask = bitor(degr_mask, bitshift(uint32(1), 7));
end

== matlab function SupervisorB1/Process B2 masks ==
  data: crit_mask_b2 input; stop_required output; degr_mask_b2 input; degraded_required output
function [stop_required, degraded_required] = ...
    preprocessB2MaskInB1(crit_mask_b2, degr_mask_b2)
%#codegen

crit_mask_b2 = uint32(crit_mask_b2);
degr_mask_b2 = uint32(degr_mask_b2);

% --- bit index ---
ESP_BIT = uint32(0);
IMU_BIT = uint32(1);
RX_BIT  = uint32(2);
SUP_BIT = uint32(3);

ESP_MASK = bitshift(uint32(1), ESP_BIT);
IMU_MASK = bitshift(uint32(1), IMU_BIT);
RX_MASK  = bitshift(uint32(1), RX_BIT);
SUP_MASK = bitshift(uint32(1), SUP_BIT);

% --- STOP: solo fault fisici ---
hard_stop_mask = bitor(ESP_MASK, IMU_MASK);
stop_required = (bitand(crit_mask_b2, hard_stop_mask) ~= 0);

% --- DEGRADED ---
rx_critical  = (bitand(crit_mask_b2, RX_MASK)  ~= 0);
sup_critical = (bitand(crit_mask_b2, SUP_MASK) ~= 0);
any_degraded = (degr_mask_b2 ~= 0);

degraded_required = rx_critical || sup_critical || any_degraded;
